simulink model "phxex_sim_swingover"  (R2025b)
settings: Solver=FixedStepDiscrete  StartTime=0.0  StopTime=14.85  FixedStep=0.004  RelTol=1e-3
values from neighbouring files (symbols this model uses):
  Trolley = phx.Body("Type", "kinematic", "Position", [xStart 0 zPivot + 0.08],          "Shape", {"Box", "Size", [0.3 0.2 0.16], "Color", [0.85 0.5 0.15]},          "Name", "Trolley")    [model_swingover.m]
undefined symbols (not defined in the file or in its folder): dspblkCoreblockFVToolHelper, gcbh
libraries: PhxLibrary x1
settings Model: Creator=lzhan  LastModifiedBy=lzhan
settings DataIOCC: SaveOutput=off  SaveTime=off
settings DebuggingCC: UnderspecifiedInitializationDetection=Classic  MergeDetectMultiDrivingBlocksExec=none
settings ModelReferenceCC: PropagateSignalLabelsOutOfModel=off

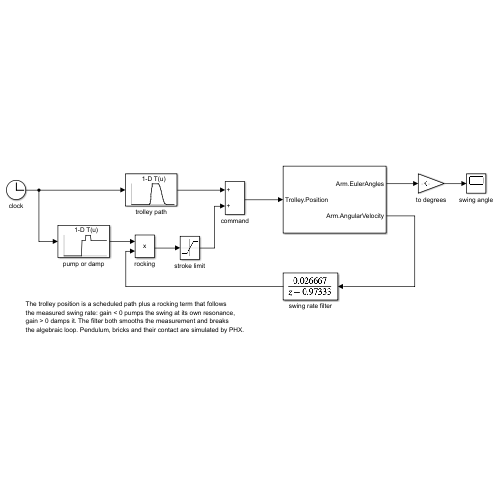
[thumbnail: Simulink's stored preview of the top-level diagram]
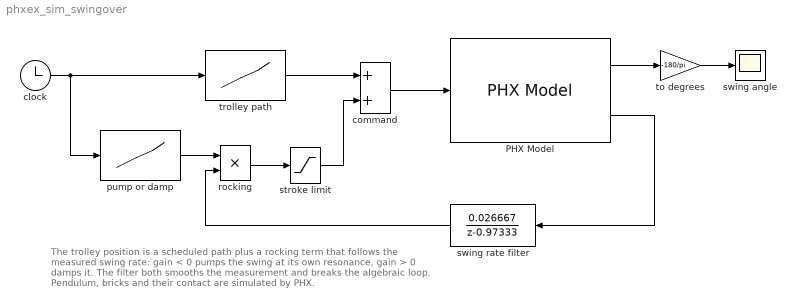
== system phxex_sim_swingover ==
  note: The trolley position is a scheduled path plus a rocking term that follows
      | the measured swing rate: gain < 0 pumps the swing at its own resonance,
      | gain > 0 damps it. The filter both smooths the measurement and breaks
      | the algebraic loop. Pendulum, bricks and their contact are simulated by PHX.
  PHX Model : PhxLibrary/PHX Model  ModelSource=saved_swingover.mat  InputRefs=Trolley.Position(1)  OutputRefs=|  ShowViewer=on  RenderEach=on  CameraPosition=[-3.3,-4.3,1.7]  CameraTarget=[-0.2,0,0.7]  SimulationStep=0.008  SimpleIcon=off  Substeps=1  CameraResolution=[0 0]
      | Arm.EulerAngles(2)
      | Arm.AngularVelocity(2)
      settings: SourceProductName=PHX Toolbox
  clock : Clock
  command : Sum
  pump or damp : Lookup_n-D  NumberOfTableDimensions=1  BreakpointsForDimension1=[0 6.45 6.75 7.85 8.15 9.85 10.15 15.85]  Table=[-0.15 -0.15 0 0 0.05 0.05 0 0]  InternalRulePriority=Speed  RndMeth=Simplest
  rocking : Product
  stroke limit : Saturate  UpperLimit=0.15  LowerLimit=-0.15
  swing angle : Scope
  swing rate filter : DiscreteTransferFcn  LoadFcn=dspblkCoreblockFVToolHelper(gcbh,'load');  Numerator=[0 0.026667]  Denominator=[1 -0.97333]  SampleTime=0.004
      settings: CopyFcn=dspblkCoreblockFVToolHelper(gcbh,'copy');  DeleteFcn=dspblkCoreblockFVToolHelper(gcbh,'close');  ModelCloseFcn=dspblkCoreblockFVToolHelper(gcbh,'close');  PreSaveFcn=dspblkCoreblockFVToolHelper(gcbh,'presave');  PostSaveFcn=dspblkCoreblockFVToolHelper(gcbh,'postsave');  CloseFcn=dspblkCoreblockFVToolHelper(gcbh,'close');
  to degrees : Gain  Gain=-180/pi
  trolley path : Lookup_n-D  NumberOfTableDimensions=1  BreakpointsForDimension1=[0 6.75 6.8417 6.9333 7.025 7.1167 7.2083 7.3 7.3917 7.4833 7.575 7.6667 7.7583 7.85 9.85 10.1 10.35 10.6 10.85 11.1 11.35 11.6 11.85 12.1 12.35 12.6 12.85 15.85]  Table=[-1.4 -1.4 -1.3523 -1.2124 -0.98995 -0.7 -0.36235 -2.2204e-16 0.36235 0.7 0.98995 1.2124 1.3523 1.4 1.4 1.3523 1.2124 0.98995 0.7 0.36235 2.2204e-16 -0.36235 -0.7 -0.98995 -1.2124 -1.3523 -1.4 -1.4]  InternalRulePriority=Speed  RndMeth=Simplest
  wires:
  clock/1 -> pump or damp/1, trolley path/1
  swing rate filter/1 -> rocking/2
  pump or damp/1 -> rocking/1
  rocking/1 -> stroke limit/1
  stroke limit/1 -> command/2
  trolley path/1 -> command/1
  command/1 -> PHX Model/1
  to degrees/1 -> swing angle/1
  PHX Model/2 -> swing rate filter/1
  PHX Model/1 -> to degrees/1
